simulink model "lab3_prob2_given"  (R2024a)
settings: Solver=VariableStepAuto  StartTime=0.0  StopTime=20  RelTol=1e-3
values from neighbouring files (symbols this model uses):
  G_den1 = [1 0 0]    [Problem2_Aldovino_Bejasa.m]
  G_den2 = [1 1]    [Problem2_Aldovino_Bejasa.m]
  G_den3 = [1 0]    [Problem2_Aldovino_Bejasa.m]
  G_den4 = [0 2 0]    [Problem2_Aldovino_Bejasa.m]
  G_num1 = [1]    [Problem2_Aldovino_Bejasa.m]
  G_num2 = [1]    [Problem2_Aldovino_Bejasa.m]
  G_num3 = [1]    [Problem2_Aldovino_Bejasa.m]
  G_num4 = [1]    [Problem2_Aldovino_Bejasa.m]
  H_den1 = [1 0]    [Problem2_Aldovino_Bejasa.m]
  H_den2 = [1 -1]    [Problem2_Aldovino_Bejasa.m]
  H_den3 = [1 -2]    [Problem2_Aldovino_Bejasa.m]
  H_num1 = [1]    [Problem2_Aldovino_Bejasa.m]
  H_num2 = [1]    [Problem2_Aldovino_Bejasa.m]
  H_num3 = [1]    [Problem2_Aldovino_Bejasa.m]
settings Model: Creator=HUAWEI  LastModifiedBy=HUAWEI

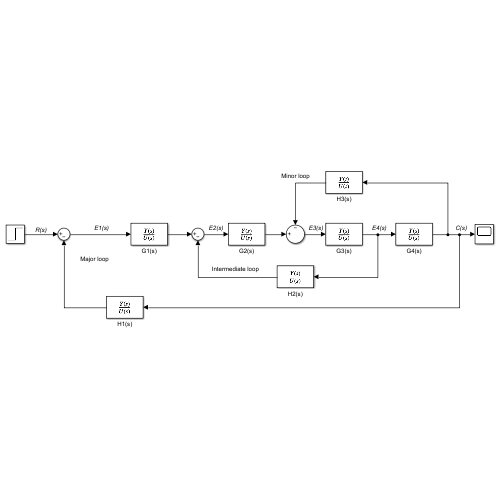
[thumbnail: Simulink's stored preview of the top-level diagram]
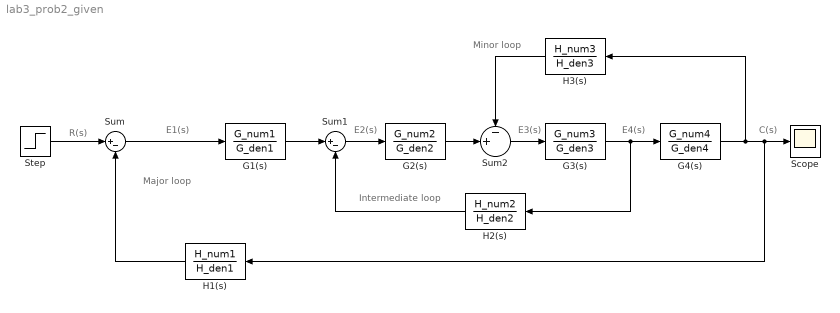
== system lab3_prob2_given ==
  note: Major loop
  note: C(s)
  note: Minor loop
  note: E4(s)
  note: E1(s)
  note: E3(s)
  note: Intermediate loop
  note: R(s)
  note: E2(s)
  G1(s) : TransferFcn  Numerator=G_num1  Denominator=G_den1
  G2(s) : TransferFcn  Numerator=G_num2  Denominator=G_den2
  G3(s) : TransferFcn  Numerator=G_num3  Denominator=G_den3
  G4(s) : TransferFcn  Numerator=G_num4  Denominator=G_den4
  H1(s) : TransferFcn  Numerator=H_num1  Denominator=H_den1
  H2(s) : TransferFcn  Numerator=H_num2  Denominator=H_den2
  H3(s) : TransferFcn  Numerator=H_num3  Denominator=H_den3
  Scope : Scope
  Step : Step  Time=0  SampleTime=0
  Sum : Sum  Inputs=|+-
  Sum1 : Sum  Inputs=|+-
  Sum2 : Sum  Inputs=-+|
  wires:
  H1(s)/1 -> Sum/2
  H3(s)/1 -> Sum2/1
  Sum1/1 -> G2(s)/1
  Sum2/1 -> G3(s)/1
  G1(s)/1 -> Sum1/1
  H2(s)/1 -> Sum1/2
  G2(s)/1 -> Sum2/2
  G4(s)/1 -> H1(s)/1, Scope/1, H3(s)/1
  Step/1 -> Sum/1
  Sum/1 -> G1(s)/1
  G3(s)/1 -> H2(s)/1, G4(s)/1
